simulink model "Proj4WBenzModel"  (R2023b)
settings: Solver=VariableStepAuto  StartTime=0.0  StopTime=1000  FixedStep=0.01  RelTol=1e-3
values from neighbouring files (symbols this model uses):
  batData_C = 150    [P4init.m]
  batData_numParallel = 74    [P4init.m]
  batData_numSeries = 96    [P4init.m]
  batData_OCV = [0, 3.1, 3.55, 3.68, 3.74, 3.76, 3.78, 3.85, 3.9, 3.95, 4.08, 4.15]    [P4init.m]
  batData_Rint = 0.1695    [P4init.m]
  batData_SOC = [0, 0.01, 0.1, 0.2, 0.3, 0.4, 0.5, 0.6, 0.7, 0.8, 0.9, 1]    [P4init.m]
  carData_C0 = 0.0041    [P4init.m]
  carData_C1 = 0.000066    (= 6.6e-05)    [P4init.m]
  carData_C2 = 0.5*Rho*A*Cd    (= 0.51156)    [P4init.m]
  carData_Calpha_f = 40000    [P4init.m]
  carData_Calpha_r = 40000    [P4init.m]
  carData_FDG = 2.5    [P4init.m]
  carData_Fyfmax = 40000*1/180*pi    (= 698.131700798)    [P4init.m]
  carData_Fyrmax = 40000*1/180*pi    (= 698.131700798)    [P4init.m]
  carData_Inertia = 1600    [P4init.m]
  carData_init_omega0 = 0    [P4init.m]
  carData_init_psi0 = 0    [P4init.m]
  carData_init_vy0 = 0    [P4init.m]
  carData_init_X0 = 0    [P4init.m]
  carData_init_Y0 = 0    [P4init.m]
  carData_Iw = 0.5*7*(carData_r^2)    (= 0.315)    [P4init.m]
  carData_lf = 1.0    (= 1)    [P4init.m]
  carData_lr = 1.5    [P4init.m]
  carData_Mass = 1000    [P4init.m]
  carData_maxAlpha = 4 / 180 * pi    (= 0.0698131700798)    [P4init.m]
  carData_r = 0.3    [P4init.m]
  carData_vxd = 15.0    (= 15)    [P4init.m]
  Cd = 0.36    [P4init.m]
  motorData_eta_speed = [0:500:10000]    [P4init.m]
  motorData_eta_torque = [0:25:325]    [P4init.m]
  motorData_eta_val = [0.740000000000000,0.740000000000000,0.740000000000000,0.740000000000000,0.740000000000000,0.740000000000000,0.740000000000000,0.740000000000000,0.740000000000000,0.740000000000000,0.740000000000000,0.740000000000000,0.740000000000000,0.740000000000000,0.740000000000000,0.740000000000000,0.740000000000000,0.740000000000000,0.740000000000000,0.740000000000000,0.740000000000000 ... (first row only)    [P4init.m]
  motorData_Inertia = 1.09    [P4init.m]
  motorData_maxtorque = [280, 280, 280, 220, 160, 110,  95,  75,  60,  55,   50,   40,     0 ... (first row only)    [P4init.m]
  motorData_rpm = [0,  1000,2000,3000,4000,5000,6000,7000,8000,9000,10000,11000, 12000]    [P4init.m]
  motorData_vbus = [350, 500, 600, 700]    [P4init.m]
  mph2mps = 1600/3600    (= 0.444444444444)    [P4init.m]
  rps2rpm = 60/(2*pi())    [P4init.m]
undefined symbols (not defined in the file or in its folder): DriveData, Time
libraries: slpidlib x1
settings Model: Creator=anshu16  LastModifiedBy=wilso
settings SolverCC: AlgebraicLoopSolver=TrustRegion
settings OptimizationCC: ReuseModelBlockBuffer=off
settings DebuggingCC: AlgebraicLoopMsg=none  UnconnectedInputMsg=warning  UnconnectedOutputMsg=warning  UnconnectedLineMsg=warning
settings ModelReferenceCC: EnableRefExpFcnMdlSchedulingChecks=on
settings SFSimCC: CustomCodeUndefinedFunction=UseInterfaceOnly

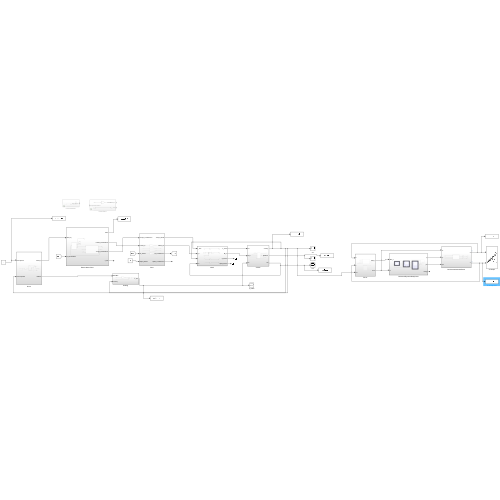
[thumbnail: Simulink's stored preview of the top-level diagram]
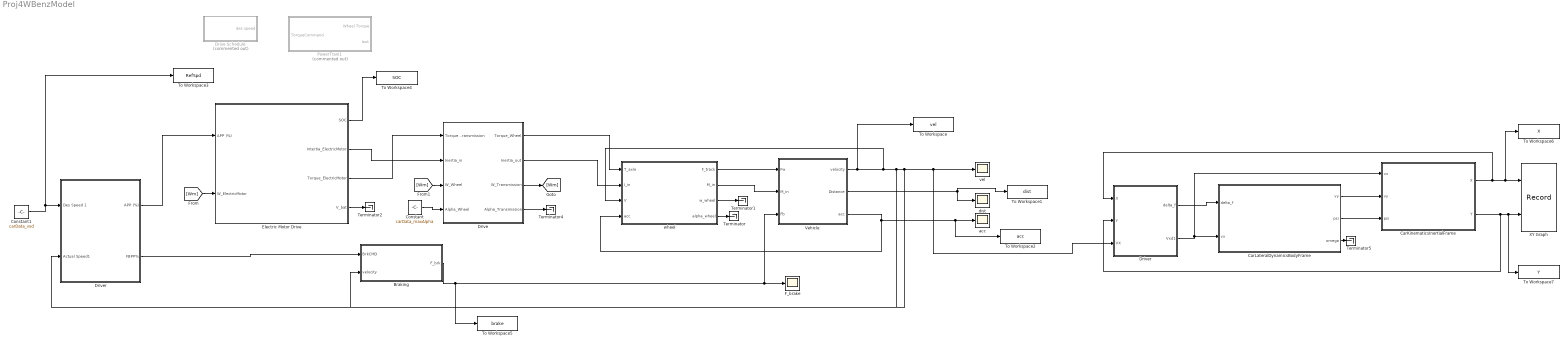
== system Proj4WBenzModel ==
  Braking : Subsystem
  CarKinematicsInertialFrame : Subsystem
  CarLateralDynamicsBodyFrame : Subsystem
  Constant : Constant  Value=carData_maxAlpha
  Constant1 : Constant  Value=carData_vxd
  Drive : Subsystem
  Drive Schedule : Subsystem  Commented=on
  Driver : Subsystem
  "Driver " : Subsystem
  Electric Motor Drive : Subsystem
  F_brake : Scope
  PowerTrain1 : Subsystem  Commented=on
  Terminator{,1..2,4..5} (5 alike) : Terminator
  To Workspace : ToWorkspace  VariableName=vel  SaveFormat=Timeseries  SampleTime=-1
  To Workspace1 : ToWorkspace  VariableName=dist  SaveFormat=Timeseries  SampleTime=-1
  To Workspace2 : ToWorkspace  VariableName=acc  SaveFormat=Timeseries  SampleTime=-1
  To Workspace3 : ToWorkspace  VariableName=RefSpd  SaveFormat=Timeseries  SampleTime=-1
  To Workspace4 : ToWorkspace  VariableName=SOC  SaveFormat=Timeseries  SampleTime=-1
  To Workspace5 : ToWorkspace  VariableName=brake  SaveFormat=Timeseries  SampleTime=-1
  To Workspace6 : ToWorkspace  VariableName=X  SaveFormat=Structure With Time  SampleTime=-1
      settings: Save2DSignal=2-D array (concatenate along first dimension)
  To Workspace7 : ToWorkspace  VariableName=Y  SaveFormat=Structure With Time  SampleTime=-1
      settings: Save2DSignal=2-D array (concatenate along first dimension)
  Vehicle : Subsystem
  XY Graph : Record  FileSettingsInternal="{\"entries\":[{\"content\":{\"excelSettings\":{\"content\":{},\"type\":\"Streamout.ExcelSettings\"}},\"type\":\"Streamout.FileSettingStorage\",\"uuid\":\"\"}],\"packageUris\":[\"http:\\/\\/schema.mathworks.com\\/mf0\\/streamout_blocks\\/R2020a\"],\"version\":\"1.0\"}"  Layout=[1 1]  SignalsInternal="{\"entries\":[{\"content\":{\"signals\":[{\"content\":{\"blockPath\":[],\"dimensions\":[1],\"domain\":\"\",\"lineColor\":\"#7e2f8e\",\"plots\":[1],\"port\":1,\"sid\":[\"\"],\"signalID\":9449,\"signalName\":\"CarKinematicsInertialFrame:1\"},\"type\":\"RecordBlkView.Signal\",\"uuid\":\"\"},{\"content\":{\"blockPath\":[],\"dimensions\":[1],\"domain\":\"\",\"lineColor\":\"#77ac30\",\"plots\":[1],\"port\":2,\"sid\":[\"\"],\"signalID\":9453,\"signalName\":\"CarKinematicsInertialFrame:2\"},\"type\":\"RecordBlkView.Signal\",\"uuid\":\"\"}]},\"type\":\"RecordBlkView.InputSignals\",\"uuid\":\"\"}],\"packageUris\":[\"http:\\/\\/schema.mathworks.com\\/mf0\\/streamout_blocks\\/R2020a\"],\"version\":\"1.0\"}"  VisualizationBindings="{\"xyplotplugin\":{\"info\":[{\"series\":[{\"bindingParametersList\":[{\"parameter\":\"X-Axis\",\"signalID\":9449,\"signalName\":\"CarKinematicsInertialFrame:1\"},{\"parameter\":\"Y-Axis\",\"signalID\":9453,\"signalName\":\"CarKinematicsInertialFrame:2\"}],\"seriesID\":25132}],\"subplotID\":1}]}}"  CompatibilityTag=XY  st=-1
  acc : Scope
  dist : Scope
  vel : Scope
  "wheel " : Subsystem
  wires:
  Braking/1("F_brk ") -> To Workspace5/1, Vehicle/3("Fb "), F_brake/1
  Vehicle/3(acc) -> "wheel "/4(acc), To Workspace2/1, acc/1
  "wheel "/2(M_in) -> Vehicle/2("M_in ")
  "wheel "/1(F_track) -> Vehicle/1("Fw ")
  Vehicle/2("Distance ") -> To Workspace1/1, dist/1
  Vehicle/1("velocity ") -> To Workspace/1, "wheel "/3(V), Braking/2("velocity "), "Driver "/2(Actual Speed1), Driver/3(VX), vel/1
  "wheel "/4(alpha_wheel) -> Terminator/1
  "wheel "/3(w_wheel) -> Terminator1/1
  Electric Motor Drive/4(V_bat) -> Terminator2/1
  Electric Motor Drive/2(Intertia_ElectricMotor) -> Drive/2(Inertia_in)
  Electric Motor Drive/3(Torque_ElectricMotor) -> Drive/1("Torque_Transmission ")
  [Wm] -> Electric Motor Drive/2(W_ElectricMotor)
  [Wm] -> Drive/3(W_Wheel)
  Drive/3(W_Transmission) -> [Wm]
  Drive/4(Alpha_Transmission) -> Terminator4/1
  "Driver "/1(APP (%)) -> Electric Motor Drive/1(APP (%))
  "Driver "/2(FBPP%) -> Braking/1("BrkCMD ")
  Drive/1(Torque_Wheel) -> "wheel "/1(T_axle)
  Drive/2(Inertia_out) -> "wheel "/2(I_in)
  Constant/1 -> Drive/4(Alpha_Wheel)
  CarLateralDynamicsBodyFrame/3(omega) -> Terminator5/1
  CarLateralDynamicsBodyFrame/1(vy) -> CarKinematicsInertialFrame/2(vy)
  CarKinematicsInertialFrame/2(Y) -> Driver/2(Y), To Workspace7/1, XY Graph/2
  Driver/2(Vxd1) -> CarKinematicsInertialFrame/1(vx), CarLateralDynamicsBodyFrame/2(vx)
  CarLateralDynamicsBodyFrame/2(psi) -> CarKinematicsInertialFrame/3(psi)
  Driver/1(delta_f) -> CarLateralDynamicsBodyFrame/1(delta_f)
  CarKinematicsInertialFrame/1(X) -> Driver/1(X), To Workspace6/1, XY Graph/1
  Constant1/1 -> To Workspace3/1, "Driver "/1(Des Speed 1)
  Electric Motor Drive/1(SOC) -> To Workspace4/1

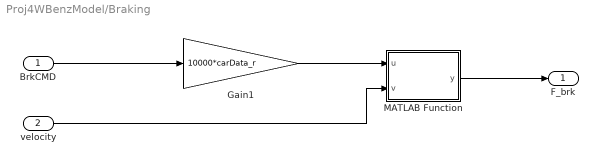
== system Proj4WBenzModel/Braking ==
  "BrkCMD " : Inport
  "velocity " : Inport  Port=2
  Gain1 : Gain  Gain=10000*carData_r
  MATLAB Function : MATLAB Function  TreatAsAtomicUnit=on
  "F_brk " : Outport  VectorParamsAs1DForOutWhenUnconnected=off
  wires:
  "BrkCMD "/1 -> Gain1/1
  Gain1/1 -> MATLAB Function/1(u)
  MATLAB Function/1(y) -> "F_brk "/1
  "velocity "/1 -> MATLAB Function/2(v)

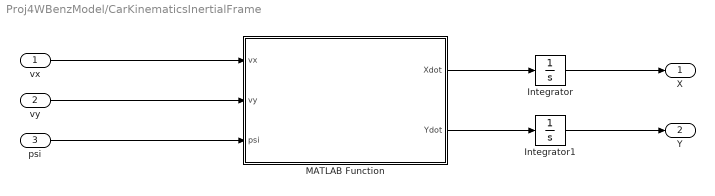
== system Proj4WBenzModel/CarKinematicsInertialFrame ==
  vx : Inport
  vy : Inport  Port=2
  psi : Inport  Port=3
  Integrator : Integrator  InitialCondition=carData_init_X0
  Integrator1 : Integrator  InitialCondition=carData_init_Y0
  MATLAB Function : MATLAB Function  TreatAsAtomicUnit=on
  X : Outport
  Y : Outport  Port=2
  wires:
  MATLAB Function/1(Xdot) -> Integrator/1
  MATLAB Function/2(Ydot) -> Integrator1/1
  Integrator/1 -> X/1
  Integrator1/1 -> Y/1
  vx/1 -> MATLAB Function/1(vx)
  vy/1 -> MATLAB Function/2(vy)
  psi/1 -> MATLAB Function/3(psi)

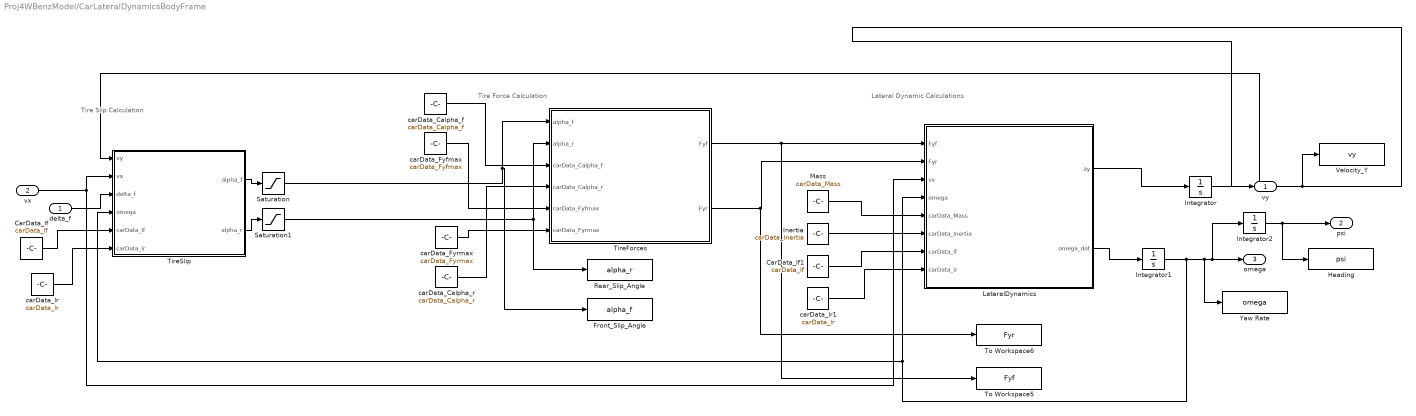
== system Proj4WBenzModel/CarLateralDynamicsBodyFrame ==
  note: Tire Slip Calculation
  note: Tire Force Calculation
  note: Lateral Dynamic Calculations
  delta_f : Inport
  vx : Inport  Port=2
  CarData_lf : Constant  Value=carData_lf
  CarData_lf1 : Constant  Value=carData_lf
  Front_Slip_Angle : ToWorkspace  VariableName=alpha_f  SaveFormat=Timeseries  SampleTime=-1
  Heading : ToWorkspace  VariableName=psi  SaveFormat=Timeseries  SampleTime=-1
  Inertia : Constant  Value=carData_Inertia
  Integrator : Integrator  InitialCondition=carData_init_vy0
  Integrator1 : Integrator  InitialCondition=carData_init_omega0
  Integrator2 : Integrator  InitialCondition=carData_init_psi0
  LateralDynamics : MATLAB Function  TreatAsAtomicUnit=on
  Mass : Constant  Value=carData_Mass
  Rear_Slip_Angle : ToWorkspace  VariableName=alpha_r  SaveFormat=Timeseries  SampleTime=-1
  Saturation : Saturate  UpperLimit=carData_maxAlpha  LowerLimit=-carData_maxAlpha
  Saturation1 : Saturate  UpperLimit=carData_maxAlpha  LowerLimit=-carData_maxAlpha
  TireForces : MATLAB Function  TreatAsAtomicUnit=on
  TireSlip : MATLAB Function  TreatAsAtomicUnit=on
  To Workspace5 : ToWorkspace  VariableName=Fyf  SaveFormat=Timeseries  SampleTime=-1
  To Workspace6 : ToWorkspace  VariableName=Fyr  SaveFormat=Timeseries  SampleTime=-1
  Velocity_Y : ToWorkspace  VariableName=vy  SaveFormat=Timeseries  SampleTime=-1
  Yaw Rate : ToWorkspace  VariableName=omega  SaveFormat=Timeseries  SampleTime=-1
  carData_Calpha_f : Constant  Value=carData_Calpha_f
  carData_Calpha_r : Constant  Value=carData_Calpha_r
  carData_Fyfmax : Constant  Value=carData_Fyfmax
  carData_Fyrmax : Constant  Value=carData_Fyrmax
  carData_lr : Constant  Value=carData_lr
  carData_lr1 : Constant  Value=carData_lr
  vy : Outport
  psi : Outport  Port=2
  omega : Outport  Port=3
  wires:
  LateralDynamics/1(ay) -> Integrator/1
  Integrator/1 -> TireSlip/1(vy), vy/1, Velocity_Y/1
  LateralDynamics/2(omega_dot) -> Integrator1/1
  Integrator1/1 -> Integrator2/1, omega/1, Yaw Rate/1, LateralDynamics/4(omega), TireSlip/4(omega)
  Saturation/1 -> TireForces/1(alpha_f), Front_Slip_Angle/1
  Saturation1/1 -> TireForces/2(alpha_r), Rear_Slip_Angle/1
  vx/1 -> LateralDynamics/3(vx), TireSlip/2(vx)
  delta_f/1 -> TireSlip/3(delta_f)
  Integrator2/1 -> Heading/1, psi/1
  TireSlip/1(alpha_f) -> Saturation/1
  TireSlip/2(alpha_r) -> Saturation1/1
  CarData_lf/1 -> TireSlip/5(carData_lf)
  carData_lr/1 -> TireSlip/6(carData_lr)
  TireForces/1(Fyf) -> To Workspace5/1, LateralDynamics/1(Fyf)
  TireForces/2(Fyr) -> To Workspace6/1, LateralDynamics/2(Fyr)
  carData_Fyfmax/1 -> TireForces/5(carData_Fyfmax)
  carData_Fyrmax/1 -> TireForces/6(carData_Fyrmax)
  carData_Calpha_f/1 -> TireForces/3(carData_Calpha_f)
  carData_Calpha_r/1 -> TireForces/4(carData_Calpha_r)
  carData_lr1/1 -> LateralDynamics/8(carData_lr)
  CarData_lf1/1 -> LateralDynamics/7(carData_lf)
  Inertia/1 -> LateralDynamics/6(carData_Inertia)
  Mass/1 -> LateralDynamics/5(carData_Mass)

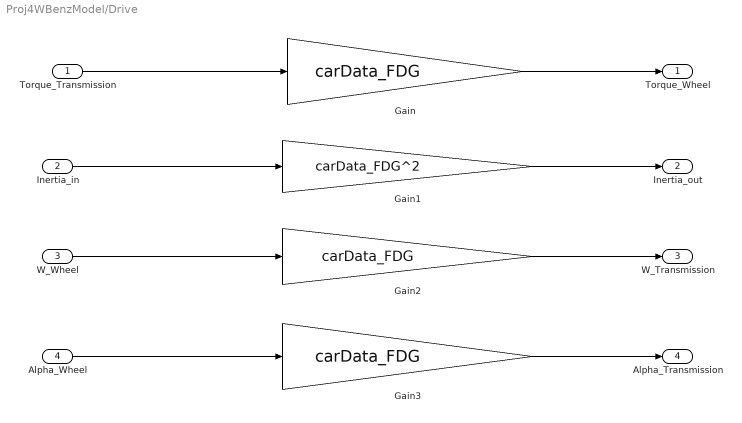
== system Proj4WBenzModel/Drive ==
  "Torque_Transmission " : Inport
  Inertia_in : Inport  Port=2
  W_Wheel : Inport  Port=3
  Alpha_Wheel : Inport  Port=4
  Gain : Gain  Gain=carData_FDG
  Gain1 : Gain  Gain=carData_FDG^2
  Gain2 : Gain  Gain=carData_FDG
  Gain3 : Gain  Gain=carData_FDG
  Torque_Wheel : Outport
  Inertia_out : Outport  Port=2
  W_Transmission : Outport  Port=3
  Alpha_Transmission : Outport  Port=4
  wires:
  "Torque_Transmission "/1 -> Gain/1
  Inertia_in/1 -> Gain1/1
  W_Wheel/1 -> Gain2/1
  Alpha_Wheel/1 -> Gain3/1
  Gain3/1 -> Alpha_Transmission/1
  Gain2/1 -> W_Transmission/1
  Gain1/1 -> Inertia_out/1
  Gain/1 -> Torque_Wheel/1

== system Proj4WBenzModel/Drive Schedule ==
  1-D Lookup Table : Lookup_n-D  NumberOfTableDimensions=1  BreakpointsForDimension1=Time  Table=DriveData  InternalRulePriority=Speed  RndMeth=Simplest
  Clock : Clock
  Gain : Gain  Gain=mph2mps
  Scope : Scope
  "des speed " : Outport  VectorParamsAs1DForOutWhenUnconnected=off
  wires:
  Clock/1 -> 1-D Lookup Table/1
  1-D Lookup Table/1 -> Gain/1
  Gain/1 -> "des speed "/1, Scope/1

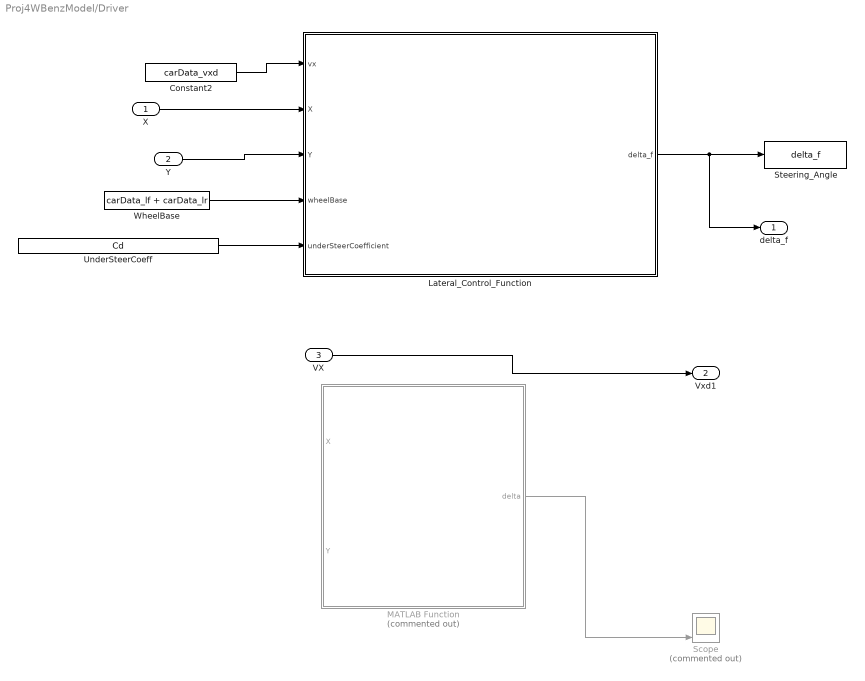
== system Proj4WBenzModel/Driver ==
  X : Inport
  Y : Inport  Port=2
  VX : Inport  Port=3
  Constant2 : Constant  Value=carData_vxd
  Lateral_Control_Function : MATLAB Function  TreatAsAtomicUnit=on
  MATLAB Function : MATLAB Function  Commented=on  TreatAsAtomicUnit=on
  Scope : Scope  Commented=on  NumInputPorts=3
  Steering_Angle : ToWorkspace  VariableName=delta_f  SaveFormat=Timeseries  SampleTime=-1
  UnderSteerCoeff : Constant  Value=Cd
  WheelBase : Constant  Value=carData_lf + carData_lr
  delta_f : Outport
  Vxd1 : Outport  Port=2
  wires:
  WheelBase/1 -> Lateral_Control_Function/4(wheelBase)
  Lateral_Control_Function/1(delta_f) -> delta_f/1, Steering_Angle/1
  UnderSteerCoeff/1 -> Lateral_Control_Function/5(underSteerCoefficient)
  MATLAB Function/1(delta) -> Scope/3
  Y/1 -> Lateral_Control_Function/3(Y)
  X/1 -> Lateral_Control_Function/2(X)
  VX/1 -> Vxd1/1
  Constant2/1 -> Lateral_Control_Function/1(vx)

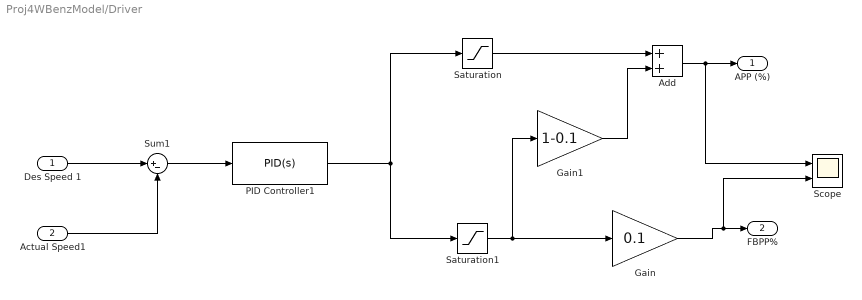
== system Proj4WBenzModel/Driver  ==
  Des Speed 1 : Inport
  Actual Speed1 : Inport  Port=2
  Add : Sum
  Gain : Gain  Gain=0.1
  Gain1 : Gain  Gain=1-0.1
  PID Controller1 : slpidlib/PID Controller  Controller=PID  Form=Parallel  TimeDomain=Continuous-time  UseExternalTs=off  SampleTime=-1  IntegratorMethod=Forward Euler  FilterMethod=Forward Euler  ControllerParametersSource=internal  P=0.1  I=0  UseKiTs=off  D=0  N=100  UseFilter=on  TunerSelectOption=Transfer Function Based (PID Tuner App)  InitialConditionSource=internal  InitialConditionForIntegrator=0  InitialConditionForFilter=0  DifferentiatorICPrevScaledInput=0  ExternalReset=none  TrackingMode=off  Kt=1  LimitOutput=on  SatLimitsSource=internal  UpperSaturationLimit=1  LowerSaturationLimit=-1  LinearizeAsGain=off  AntiWindupMode=none  Kb=1  LimitIntegrator=off  UpperIntegratorSaturationLimit=inf  LowerIntegratorSaturationLimit=-inf  POutMin=[]  POutMax=[]  IOutMin=[]  IOutMax=[]  DOutMin=[]  DOutMax=[]  NOutMin=[]  NOutMax=[]  SumOutMin=[]  SumOutMax=[]  SaturationOutMin=[]  SaturationOutMax=[]  PParamMin=[]  PParamMax=[]  IParamMin=[]  IParamMax=[]  DParamMin=[]  DParamMax=[]  NParamMin=[]  NParamMax=[]  KbParamMin=[]  KbParamMax=[]  KtParamMin=[]  KtParamMax=[]  KbOutMin=[]  KbOutMax=[]  KtOutMin=[]  KtOutMax=[]  IntegratorOutMin=[]  IntegratorOutMax=[]  FilterOutMin=[]  FilterOutMax=[]  SumI1OutMin=[]  SumI1OutMax=[]  SumI2OutMin=[]  SumI2OutMax=[]  SumI3OutMin=[]  SumI3OutMax=[]  SumI4OutMin=[]  SumI4OutMax=[]  SumDOutMin=[]  SumDOutMax=[]  DifferentiatorOutMin=[]  DifferentiatorOutMax=[]  FilterDiffOutCoefMin=[]  FilterDiffOutCoefMax=[]  ReciprocalOutMin=[]  ReciprocalOutMax=[]  SumDenOutMin=[]  SumDenOutMax=[]  SumNumOutMin=[]  SumNumOutMax=[]  DivideOutMin=[]  DivideOutMax=[]  UdiffTsProdOutMin=[]  UdiffTsProdOutMax=[]  NTsProdOutMin=[]  NTsProdOutMax=[]  UintegralTsProdOutMin=[]  UintegralTsProdOutMax=[]  UngainTsProdOutMin=[]  UngainTsProdOutMax=[]  ClampingZeroOutDataTypeStr=Inherit: Inherit via back propagation  ClampingZeroOutMin=[]  ClampingZeroOutMax=[]  FilterDenConstantOutDataTypeStr=Inherit: Inherit via back propagation  FilterDenConstantOutMin=[]  FilterDenConstantOutMax=[]  PCopyOutDataTypeStr=Inherit: Inherit via back propagation  PCopyOutMin=[]  PCopyOutMax=[]  NCopyOutDataTypeStr=Inherit: Inherit via back propagation  NCopyOutMin=[]  NCopyOutMax=[]  IntegratorContinuousStateAttributes=''  IntegratorStateMustResolveToSignalObject=off  IntegratorRTWStateStorageClass=Auto  FilterContinuousStateAttributes=''  FilterStateMustResolveToSignalObject=off  FilterRTWStateStorageClass=Auto  ParallelPVariant=InternalParameters  IdealPVariant=Disabled  IVariant=InternalParameters  DVariant=InternalParameters  IntegratorVariant=Continuous  SatVariant=Enabled  AWVariant=Passthrough  PCopyVariant=Disabled  TRVariant=Disabled  FdbkBlocksVariant=Forward  IdealPFdbkVariant=Disabled  SatFdbkVariant=Disabled  DerivativeFilterVariant=ContFilter  NVariant=InternalParameters  NCopyVariant=Disabled  FilterICVariant=InternalICsFilter  IntegratorICVariant=InternalICs  ExternalResetVariant=Disabled  TRSumVariant=Passthrough  SumFdbkVariant=Disabled  SumVariant=Sum_PID  TsampFilterVariant=InternalTs  TsampNgainVariant=Passthrough  TsampIntegralVariant=Disabled_SignalSpec  ExternalSaturationOutDataTypeStr=Inherit: Same as second input
  Saturation : Saturate
  Saturation1 : Saturate
  Scope : Scope  NumInputPorts=2
  Sum1 : Sum  Inputs=|+-
  APP (%) : Outport
  FBPP% : Outport  Port=2
  wires:
  Sum1/1 -> PID Controller1/1
  Des Speed 1/1 -> Sum1/1
  Actual Speed1/1 -> Sum1/2
  PID Controller1/1 -> Saturation1/1, Saturation/1
  Saturation/1 -> Add/1
  Saturation1/1 -> Gain1/1, Gain/1
  Gain1/1 -> Add/2
  Add/1 -> Scope/1, APP (%)/1
  Gain/1 -> Scope/2, FBPP%/1

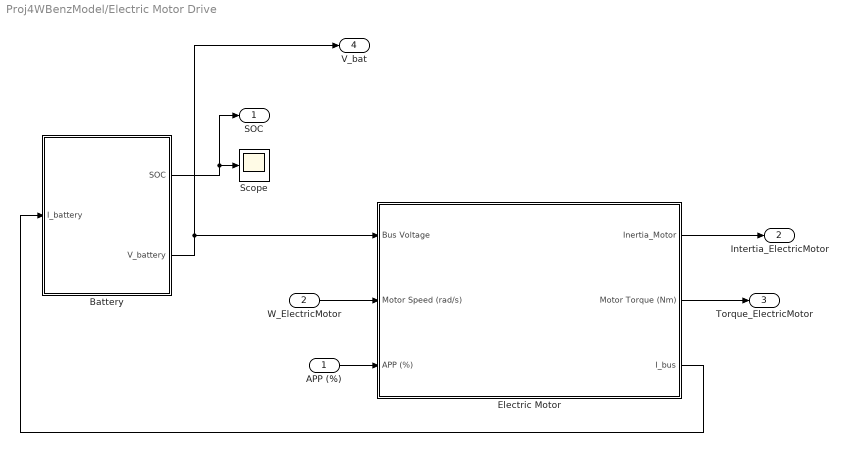
== system Proj4WBenzModel/Electric Motor Drive ==
  APP (%) : Inport
  W_ElectricMotor : Inport  Port=2
  Battery : Subsystem
  Electric Motor : Subsystem
  Scope : Scope
  SOC : Outport
  Intertia_ElectricMotor : Outport  Port=2
  Torque_ElectricMotor : Outport  Port=3
  V_bat : Outport  Port=4
  wires:
  Battery/1(SOC) -> SOC/1, Scope/1
  APP (%)/1 -> Electric Motor/3(APP (%))
  W_ElectricMotor/1 -> Electric Motor/2(Motor Speed (rad/s))
  Electric Motor/2(Motor Torque (Nm)) -> Torque_ElectricMotor/1
  Electric Motor/1(Inertia_Motor) -> Intertia_ElectricMotor/1
  Electric Motor/3(I_bus) -> Battery/1(I_battery)
  Battery/2(V_battery) -> V_bat/1, Electric Motor/1(Bus Voltage)

== system Proj4WBenzModel/PowerTrain1 ==
  TorqueCommand : Inport
  Constant : Constant  Value=0
  Gain : Gain  Gain=1500
  Wheel Torque : Outport
  Iout : Outport  Port=2
  wires:
  Constant/1 -> Iout/1
  Gain/1 -> Wheel Torque/1
  TorqueCommand/1 -> Gain/1

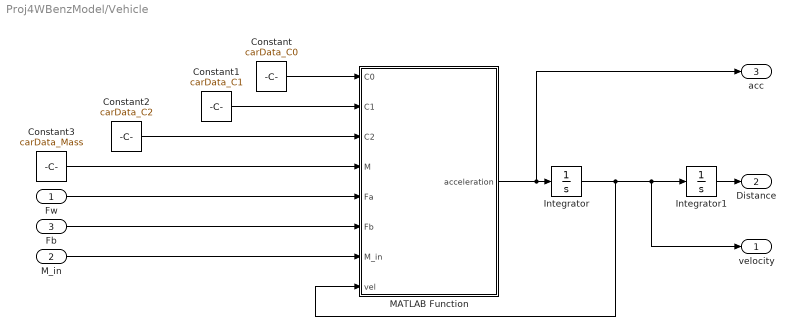
== system Proj4WBenzModel/Vehicle ==
  "Fw " : Inport
  "M_in " : Inport  Port=2
  "Fb " : Inport  Port=3
  Constant : Constant  Value=carData_C0
  Constant1 : Constant  Value=carData_C1
  Constant2 : Constant  Value=carData_C2
  Constant3 : Constant  Value=carData_Mass
  Integrator : Integrator  LimitOutput=on  LowerSaturationLimit=0
  Integrator1 : Integrator
  MATLAB Function : MATLAB Function  TreatAsAtomicUnit=on
  "velocity " : Outport  VectorParamsAs1DForOutWhenUnconnected=off
  "Distance " : Outport  Port=2  VectorParamsAs1DForOutWhenUnconnected=off
  acc : Outport  Port=3
  wires:
  Constant1/1 -> MATLAB Function/2(C1)
  Constant/1 -> MATLAB Function/1(C0)
  MATLAB Function/1(acceleration) -> acc/1, Integrator/1
  Constant2/1 -> MATLAB Function/3(C2)
  Constant3/1 -> MATLAB Function/4(M)
  "Fw "/1 -> MATLAB Function/5(Fa)
  "Fb "/1 -> MATLAB Function/6(Fb)
  Integrator/1 -> MATLAB Function/8(vel), "velocity "/1, Integrator1/1
  Integrator1/1 -> "Distance "/1
  "M_in "/1 -> MATLAB Function/7(M_in)

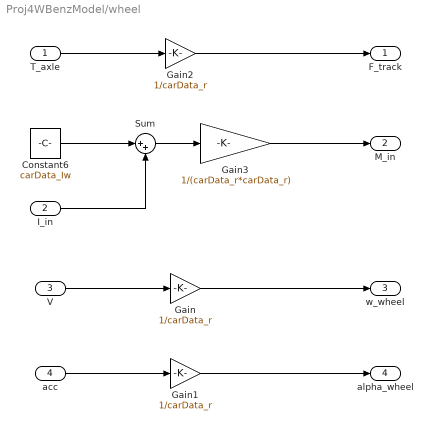
== system Proj4WBenzModel/wheel  ==
  T_axle : Inport
  I_in : Inport  Port=2
  V : Inport  Port=3
  acc : Inport  Port=4
  Constant6 : Constant  Value=carData_Iw
  Gain : Gain  Gain=1/carData_r
  Gain1 : Gain  Gain=1/carData_r
  Gain2 : Gain  Gain=1/carData_r
  Gain3 : Gain  Gain=1/(carData_r*carData_r)
  Sum : Sum  Inputs=|++
  F_track : Outport
  M_in : Outport  Port=2
  w_wheel : Outport  Port=3
  alpha_wheel : Outport  Port=4
  wires:
  Gain/1 -> w_wheel/1
  V/1 -> Gain/1
  acc/1 -> Gain1/1
  Gain1/1 -> alpha_wheel/1
  T_axle/1 -> Gain2/1
  Gain2/1 -> F_track/1
  Gain3/1 -> M_in/1
  Constant6/1 -> Sum/1
  I_in/1 -> Sum/2
  Sum/1 -> Gain3/1

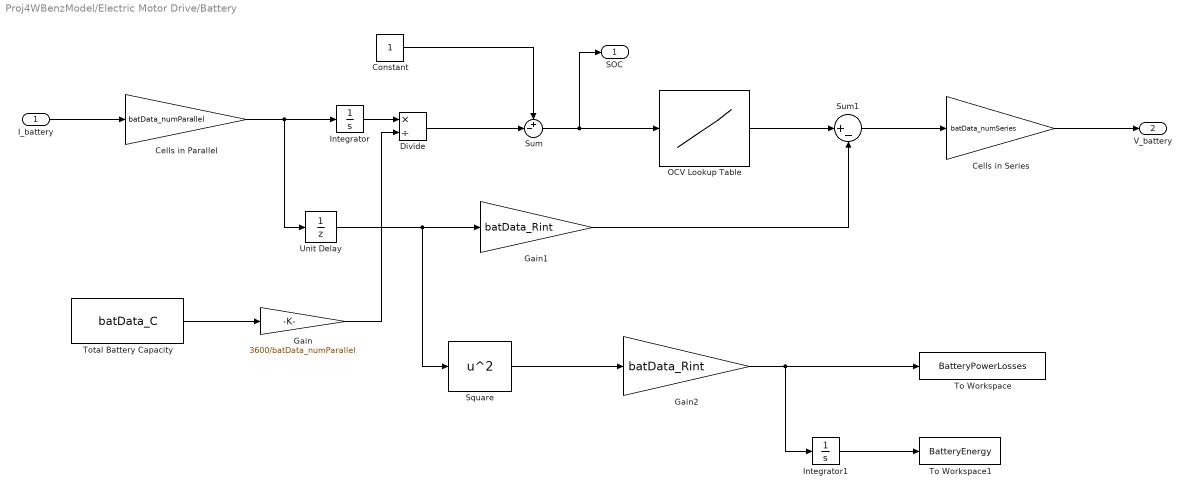
== system Proj4WBenzModel/Electric Motor Drive/Battery ==
  I_battery : Inport
  Cells in Parallel : Gain  Gain=batData_numParallel
  Cells in Series : Gain  Gain=batData_numSeries
  Constant : Constant
  Divide : Product  Inputs=*/
  Gain : Gain  Gain=3600/batData_numParallel
  Gain1 : Gain  Gain=batData_Rint
  Gain2 : Gain  Gain=batData_Rint
  Integrator : Integrator
  Integrator1 : Integrator
  OCV Lookup Table : Lookup_n-D  NumberOfTableDimensions=1  BreakpointsForDimension1=batData_SOC  BreakpointsForDimension3=[5, 7]  Table=batData_OCV  InternalRulePriority=Speed  RndMeth=Simplest
  Square : Math  Operator=square
  Sum : Sum  Inputs=+-|
  Sum1 : Sum  Inputs=|+-
  To Workspace : ToWorkspace  VariableName=BatteryPowerLosses  SaveFormat=Timeseries  SampleTime=-1
  To Workspace1 : ToWorkspace  VariableName=BatteryEnergy  SaveFormat=Timeseries  SampleTime=-1
  Total Battery Capacity : Constant  Value=batData_C
  Unit Delay : UnitDelay  SampleTime=-1  HasFrameUpgradeWarning=on
  SOC : Outport
  V_battery : Outport  Port=2
  wires:
  I_battery/1 -> Cells in Parallel/1
  Integrator/1 -> Divide/1
  Cells in Parallel/1 -> Unit Delay/1, Integrator/1
  Constant/1 -> Sum/1
  Divide/1 -> Sum/2
  Sum/1 -> OCV Lookup Table/1, SOC/1
  OCV Lookup Table/1 -> Sum1/1
  Gain/1 -> Divide/2
  Unit Delay/1 -> Square/1, Gain1/1
  Square/1 -> Gain2/1
  Cells in Series/1 -> V_battery/1
  Sum1/1 -> Cells in Series/1
  Gain1/1 -> Sum1/2
  Gain2/1 -> Integrator1/1, To Workspace/1
  Integrator1/1 -> To Workspace1/1
  Total Battery Capacity/1 -> Gain/1

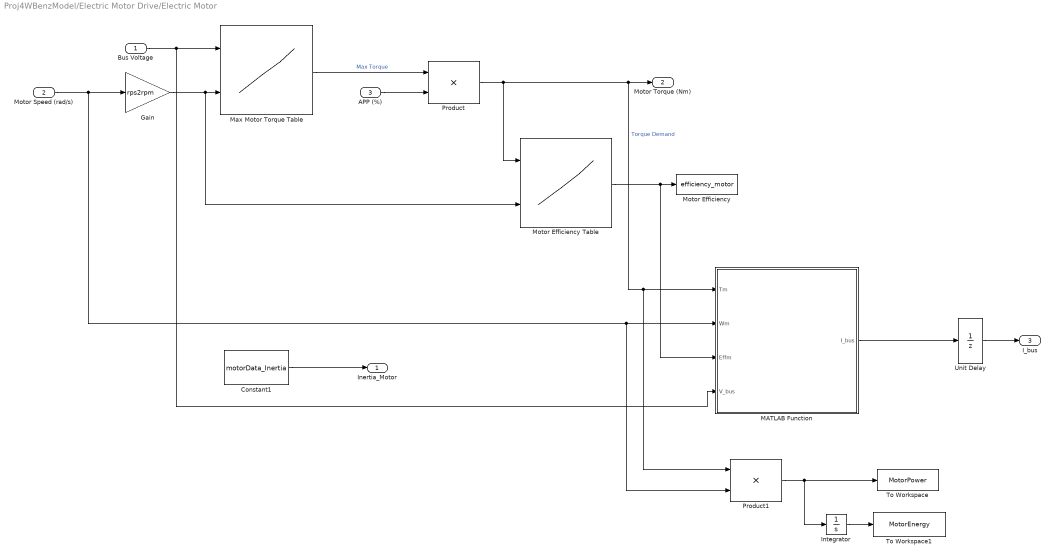
== system Proj4WBenzModel/Electric Motor Drive/Electric Motor ==
  Bus Voltage : Inport
  Motor Speed (rad/s) : Inport  Port=2
  APP (%) : Inport  Port=3
  Constant1 : Constant  Value=motorData_Inertia
  Gain : Gain  Gain=rps2rpm
  Integrator : Integrator
  MATLAB Function : MATLAB Function  TreatAsAtomicUnit=on
  Max Motor Torque Table : Lookup_n-D  BreakpointsForDimension1=motorData_vbus  BreakpointsForDimension2=motorData_rpm  BreakpointsForDimension3=[5, 7]  Table=motorData_maxtorque  InternalRulePriority=Speed  RndMeth=Simplest
      settings: InputPortMap=u0,u1
  Motor Efficiency : ToWorkspace  VariableName=efficiency_motor  SaveFormat=Timeseries  SampleTime=-1
  Motor Efficiency Table : Lookup_n-D  BreakpointsForDimension1=motorData_eta_torque  BreakpointsForDimension2=motorData_eta_speed  BreakpointsForDimension3=[5, 7]  Table=motorData_eta_val  InternalRulePriority=Speed  RndMeth=Simplest
      settings: InputPortMap=u0,u1
  Product : Product
  Product1 : Product
  To Workspace : ToWorkspace  VariableName=MotorPower  SaveFormat=Timeseries  SampleTime=-1
  To Workspace1 : ToWorkspace  VariableName=MotorEnergy  SaveFormat=Timeseries  SampleTime=-1
  Unit Delay : UnitDelay  SampleTime=-1  HasFrameUpgradeWarning=on
  Inertia_Motor : Outport
  Motor Torque (Nm) : Outport  Port=2
  I_bus : Outport  Port=3
  wires:
  Bus Voltage/1 -> MATLAB Function/4(V_bus), Max Motor Torque Table/1
  Gain/1 -> Motor Efficiency Table/2, Max Motor Torque Table/2
  Motor Speed (rad/s)/1 -> Product1/2, MATLAB Function/2(Wm), Gain/1
  Motor Efficiency Table/1 -> MATLAB Function/3(Effm), Motor Efficiency/1
  Constant1/1 -> Inertia_Motor/1
  Max Motor Torque Table/1 -> Product/1  "Max Torque"
  APP (%)/1 -> Product/2
  Product/1 -> Motor Efficiency Table/1, Product1/1, MATLAB Function/1(Tm), Motor Torque (Nm)/1  "Torque Demand"
  MATLAB Function/1(I_bus) -> Unit Delay/1
  Unit Delay/1 -> I_bus/1
  Product1/1 -> Integrator/1, To Workspace/1
  Integrator/1 -> To Workspace1/1

== matlab function Proj4WBenzModel/Driver/MATLAB Function ==
  data: X input; delta output; Y input
function delta = SimplestDriver(X,Y)

%===============================
% if abs(Y)<0.5
%     delta = 0;
% elseif abs(Y - 400) < 0.5
%     delta = 0;
% elseif X > 900
%     delta = 5;
% else
%     delta = -5;
% end



%===============================
% if X > 900
%     delta = 5;
% elseif X < 0
%     delta = -5;
% else
%     delta = 0;
% end

%===============================
if X > 900
    delta = 5;
elseif X < 0
    delta = 5;
else
    delta = 0;
end

== matlab function Proj4WBenzModel/CarKinematicsInertialFrame/MATLAB Function ==
  data: vx input; Xdot output; vy input; psi input; Ydot output
function [Xdot, Ydot] = carKinematicsInertiaFrame(vx, vy, psi)
    % Transform body frame velocities to inertial frame
    Xdot = vx * cos(psi) - vy * sin(psi);
    Ydot = vx * sin(psi) + vy * cos(psi);
end

== matlab function Proj4WBenzModel/Vehicle/MATLAB Function ==
  data: C0 input; acceleration output; C1 input; C2 input; M input; Fa input; Fb input; M_in input; vel input
function acceleration   = vehicle(C0,C1,C2,M,Fa,Fb,M_in, vel)

acceleration = (((Fa-Fb))-(C0+ C1*vel + C2*(vel)^2))/(M+M_in);

== matlab function Proj4WBenzModel/Electric Motor Drive/Electric Motor/MATLAB Function ==
  data: Tm input; I_bus output; Wm input; Effm input; V_bus input
function I_bus = fnc(Tm,Wm, Effm, V_bus)

    Pm = Tm*Wm;
    sgn_m = Pm / (abs(Pm) + 0.001);
    Pe = Pm * (Effm^sgn_m);
    I_bus = Pe/V_bus;

== matlab function Proj4WBenzModel/CarLateralDynamicsBodyFrame/LateralDynamics ==
  data: Fyf input; ay output; Fyr input; vx input; omega input; carData_Mass input; carData_Inertia input; carData_lf input; carData_lr input; omega_dot output
function [ay, omega_dot] = lateralDynamics(Fyf, Fyr, vx, omega, carData_Mass, carData_Inertia, carData_lf, carData_lr)
    % Calculate lateral acceleration
    ay = (Fyf + Fyr) / carData_Mass;

    % Calculate the rate of change of yaw rate
    omega_dot = (Fyf * carData_lf - Fyr * carData_lr) / carData_Inertia;
end

== matlab function Proj4WBenzModel/CarLateralDynamicsBodyFrame/TireForces ==
  data: Fyf output; Fyr output; alpha_f input; alpha_r input; carData_Calpha_f input; carData_Calpha_r input; carData_Fyfmax input; carData_Fyrmax input
function [Fyf, Fyr] = tireForces(alpha_f, alpha_r, carData_Calpha_f, carData_Calpha_r, carData_Fyfmax, carData_Fyrmax)

    % Calculate the potential front and rear lateral tire forces
    potentialFyf = -carData_Calpha_f * alpha_f;
    potentialFyr = -carData_Calpha_r * alpha_r;

    % Saturate the tire forces to the maximum limits
    Fyf = max(min(potentialFyf, carData_Fyfmax), -carData_Fyfmax);
    Fyr = max(min(potentialFyr, carData_Fyrmax), -carData_Fyrmax);

end

== matlab function Proj4WBenzModel/CarLateralDynamicsBodyFrame/TireSlip ==
  data: vy input; alpha_f output; vx input; delta_f input; omega input; alpha_r output; carData_lf input; carData_lr input
function [alpha_f, alpha_r] = fcn(vy, vx, delta_f, omega, carData_lf, carData_lr)
    alpha_f = atan2((vy + carData_lf * omega), vx) - delta_f;
    alpha_r = atan2((vy - carData_lr * omega), vx);
end

== matlab function Proj4WBenzModel/Braking/MATLAB Function ==
  data: u input; y output; v input
function y = fcn(u,v)
%y =u*sign(v)
y = u * v/(abs(v)+0.001);
y = u;

== matlab function Proj4WBenzModel/Driver/Lateral_Control_Function ==
  data: vx input; delta_f output; X input; Y input; wheelBase input; underSteerCoefficient input
function delta_f   = latControl(vx,X,Y,wheelBase, underSteerCoefficient)

track_radius = 200;
track_length = 900;

track_seg1_x0 = 0;
track_seg1_y0 = 0;
track_seg1_x1 = track_length;
track_seg1_y1 = 0;
track_seg2_x0 = track_seg1_x1;
track_seg2_y0 = track_seg1_y1;
track_seg2_x1 = track_seg2_x0;
track_seg2_y1 = track_seg2_y0 + 2 * track_radius;
track_seg3_x0 = track_seg2_x1;
track_seg3_y0 = track_seg2_y1;
track_seg3_x1 = track_seg3_x0 - track_length;
track_seg3_y1 = track_seg3_y0;
track_seg4_x0 = track_seg3_x1;
track_seg4_y0 = track_seg3_y1;
track_seg4_x1 = track_seg1_x0;
track_seg4_y1 = track_seg1_y0;

if X > track_seg1_x0
    if X > track_seg1_x1
        segment = 2;
    else
        if Y > (track_seg2_y0 + track_seg2_y1)/2
            segment = 3;
        else
            segment = 1;
        end
    end
else
    segment = 4;
end



switch(segment)
    case 1
        delta_f = 0;
    case 2
        delta_f = - (wheelBase / track_radius + 1 * underSteerCoefficient * vx^2);
    case 3
        delta_f = 0;
    case 4
        delta_f = - (wheelBase / track_radius + 1 * underSteerCoefficient * vx^2);
    otherwise
        delta_f = 0;
end
